simulink model "Motion_planner_Street_Drone"  (R2019b)
settings: Solver=FixedStepAuto  StartTime=0.0  StopTime=25  FixedStep=0.0075  MaxStep=1e-1  MinStep=1e-3  RelTol=1e-3  AbsTol=1e-4
InitFcn:
  | SD_init1
values from neighbouring files (symbols this model uses):
  cost = [2.71432892747 3.32441927977 3.79268757264 4.85642115368 6.12135035287 7.09825974303 9.57278659789 1.55754789407 1.51399555616 2.57723707661 3.8468529147 4.8336387623 ... (2430 elements, 1x2430)]    [matlab.mat]
  Front_brake = [0 2.2085352751 4.15209150797 6.12733711785 8.16604105928 9.79119154879 12.1808659635 14.1242630413 16.1155522836 18.1386900579 20.0839213981 22.1313006548 ... (68 elements, 34x2)]    [Front_brake.mat]
  N = size(X,1)    [curvature.m]
  obsx = [dx1 dx2 dx3 dx4]'    [dynamic_collison.m]    (also in dynamic_detection1.m = [x1 x2 x3 x4]')
  obsy = [dy1 dy2 dy3 dy4]'    [dynamic_collison.m]    (also in dynamic_detection1.m = [y1 y2 y3 y4]')
  x = obs_path(i,1)    [dynamic_collison.m]    (also in dynamic_detection1.m)
  X = [X]    [curvature.m]
  y = obs_path(i,2)    [dynamic_collison.m]    (also in dynamic_detection1.m)
undefined symbols (not defined in the file or in its folder): d, dfin, dini, Ki, Kp, L_0f, lookahead_time, lookahead_time_rev, Rear_brake, sigbuilder_block, steer_ratio, steer_sens, tfin, tini, TPS_0, xfin, Y, yfin, Z
libraries: sm_lib x290, nesl_utility x136, simulink x6, vrlib x2, powerlib_meascontrol x2
(part 13 of 14)

== system Motion_planner_Street_Drone/Trajectory Tracker/KM- StreetDrone/Street_Drone/Vehicle/RR_Wheel/For Validation ==
  Inputs : Inport
  Derivative : Derivative
  Integrator : Integrator
  Selector : Selector  InputPortWidth=40  IndexOptions=Index vector (dialog)  Indices=[3]  OutputSizes=1
  Selector1 : Selector  InputPortWidth=40  IndexOptions=Index vector (dialog)  Indices=[2]  OutputSizes=1
  Selector10 : Selector  InputPortWidth=40  IndexOptions=Index vector (dialog)  Indices=[28]  OutputSizes=1
  Selector11 : Selector  InputPortWidth=40  IndexOptions=Index vector (dialog)  Indices=[13]  OutputSizes=1
  Selector12 : Selector  InputPortWidth=40  IndexOptions=Index vector (dialog)  Indices=[5]  OutputSizes=1
  Selector2 : Selector  InputPortWidth=40  IndexOptions=Index vector (dialog)  Indices=[7]  OutputSizes=1
  Selector3 : Selector  InputPortWidth=40  IndexOptions=Index vector (dialog)  Indices=[1]  OutputSizes=1
  Selector4 : Selector  InputPortWidth=40  IndexOptions=Index vector (dialog)  Indices=[8]  OutputSizes=1
  Selector5 : Selector  InputPortWidth=40  IndexOptions=Index vector (dialog)  Indices=[11]  OutputSizes=1
  Selector6 : Selector  InputPortWidth=40  IndexOptions=Index vector (dialog)  Indices=[16]  OutputSizes=1
  Selector7 : Selector  InputPortWidth=40  IndexOptions=Index vector (dialog)  Indices=[17]  OutputSizes=1
  Selector8 : Selector  InputPortWidth=40  IndexOptions=Index vector (dialog)  Indices=[18]  OutputSizes=1
  Selector9 : Selector  InputPortWidth=40  IndexOptions=Index vector (dialog)  Indices=[24]  OutputSizes=1
  tag scope: RR_Fx=global, RR_Fy=global, RR_Fz=global, RR_Kappa=global, RR_My=global, RR_Re=global, RR_Vx=global, RR_alfa=global, RR_ax=global, RR_distance=global, RR_mu_x=global, RR_mu_y=global, RR_psi=global, RR_psidot=global, RR_tp=global
  wires:
  Selector12/1 -> [RR_My]
  Derivative/1 -> [RR_ax]
  Integrator/1 -> [RR_psi]
  Selector10/1 -> [RR_distance]
  Selector9/1 -> [RR_psidot], Integrator/1
  Selector8/1 -> [RR_mu_y]
  Selector7/1 -> [RR_mu_x]
  Selector6/1 -> [RR_tp]
  Selector5/1 -> [RR_Vx], Derivative/1
  Selector4/1 -> [RR_alfa]
  Selector3/1 -> [RR_Fx]
  Selector2/1 -> [RR_Kappa]
  Selector1/1 -> [RR_Fy]
  Selector/1 -> [RR_Fz]
  Selector11/1 -> [RR_Re]
  Inputs/1 -> Selector4/1, Selector2/1, Selector/1, Selector1/1, Selector3/1, Selector12/1, Selector5/1, Selector11/1, Selector6/1, Selector7/1, Selector8/1, Selector9/1, Selector10/1

== system Motion_planner_Street_Drone/Trajectory Tracker/KM- StreetDrone/Street_Drone/Vehicle/RR_Wheel/Non-moving road ==
  omega2 : Constant  Value=zeros(18,1)
  road : Outport
  wires:
  omega2/1 -> road/1

== system Motion_planner_Street_Drone/Trajectory Tracker/KM- StreetDrone/Street_Drone/Vehicle/RR_Wheel/Scaling factors ==
  s_LKX : Constant  Value=LKX
  s_LKY : Constant  Value=LKY
  s_LKYC : Constant  Value=LKYC
  s_LKZC : Constant  Value=LKZC
  s_LMUX : Constant  Value=LMUX
  s_LMUY : Constant  Value=LMUY
  s_LTR : Constant  Value=LTR
  scaling_vector : Mux  Inputs=7
  scaling : Outport
  wires:
  s_LMUX/1 -> scaling_vector/1
  s_LKX/1 -> scaling_vector/2
  s_LMUY/1 -> scaling_vector/3
  s_LKY/1 -> scaling_vector/4
  s_LKYC/1 -> scaling_vector/5
  s_LTR/1 -> scaling_vector/6
  s_LKZC/1 -> scaling_vector/7
  scaling_vector/1 -> scaling/1

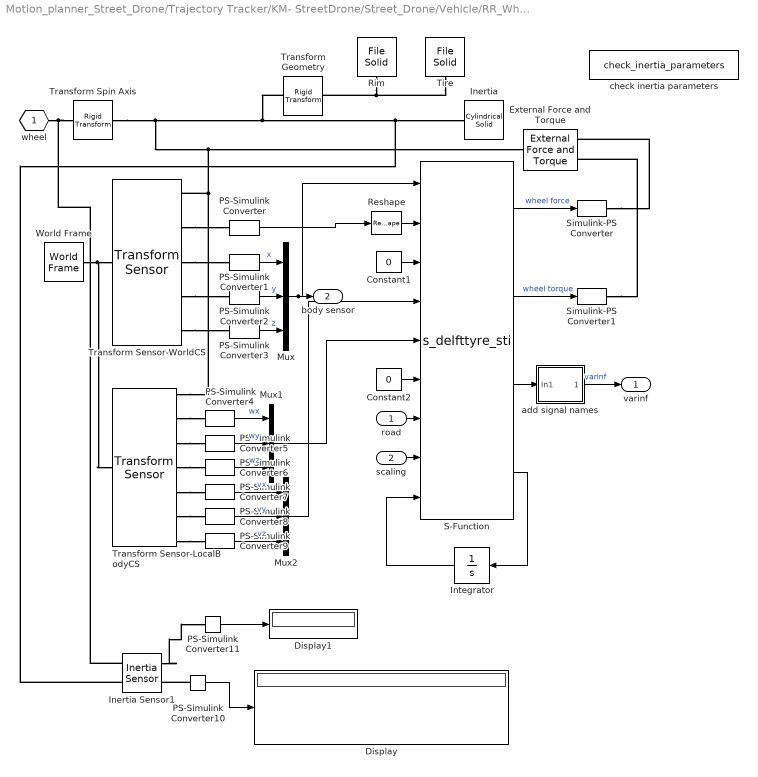
== system Motion_planner_Street_Drone/Trajectory Tracker/KM- StreetDrone/Street_Drone/Vehicle/RR_Wheel/SimMechanics2G Wheel + tyre ==
  road : Inport
  scaling : Inport  Port=2
  Constant1 : Constant  Value=0
  Constant2 : Constant  Value=0
  Display : Display
  Display1 : Display
  External Force and Torque : sm_lib/Forces and Torques/External Force and Torque  ForceResolutionFrame=AttachedFrame  EnableForceX=off  EnableForceY=off  EnableForceZ=off  EnableForce=on  TorqueResolutionFrame=AttachedFrame  EnableTorqueX=off  EnableTorqueY=off  EnableTorqueZ=off  EnableTorque=on
  Inertia : sm_lib/Body Elements/Cylindrical Solid  GraphicAmbientColor=[0.15 0.15 0.15 1.0]  BasedOnType=Density  CenterOfMass=[0 0 0]  CenterOfMassUnits=m  GraphicDiffuseColor=[0.2 0.8 1.0]  CylinderLength=0.001  CylinderLengthUnits=m  CylinderRadius=0.001  CylinderRadiusUnits=m  Density=1000  DensityUnits=kg/(m^3)  DoExposeReferenceFrame=on  GraphicEmissiveColor=[0.0 0.0 0.0 1.0]  ExportEntireGeometry=off  SerializedFrames=<Frames/>  MarkerShape=Sphere  MarkerSize=10  GraphicType=FromGeometry  InertiaType=Custom  Mass=mass  MassUnits=kg  MomentsOfInertia=[Imat(1,1) Imat(2,2) Imat(3,3)]  MomentsOfInertiaUnits=kg*m^2  GraphicOpacity=1.0  ProductsOfInertia=[0 0 0]  ProductsOfInertiaUnits=kg*m^2  GraphicShininess=75  GraphicSpecularColor=[0.5 0.5 0.5 1.0]  GraphicVisPropType=SimpleVisualProperties
  Inertia Sensor1 : sm_lib/Body Elements/Inertia Sensor  SensorExtent=BodyGroup  SpanWeldJoints=off  ExcludeGroundedBodies=off  MeasurementFrame=Custom  SenseMass=on  SenseCenterOfMass=off  SenseInertiaMatrix=on  SenseCenteredInertiaMatrix=off  SensePrincipalInertiaMatrix=off  SenseRotationMatrix=off  GraphicType=PrincipalInertiaFrame  PrincipalInertiaFrameSize=20  GraphicVisPropType=SimpleVisualProperties  GraphicDiffuseColor=[0.5 0.5 0.5]  GraphicSpecularColor=[0.5 0.5 0.5 1.0]  GraphicAmbientColor=[0.15 0.15 0.15 1.0]  GraphicEmissiveColor=[0.0 0.0 0.0 1.0]  GraphicShininess=75  GraphicOpacity=1.0
      settings: SourceProductBaseCode=MS
  Integrator : Integrator  InitialCondition=zeros(1,40)
  Mux : Mux  Inputs=3
  Mux1 : Mux  Inputs=3
  Mux2 : Mux  Inputs=3
  PS-Simulink Converter{,1..9} (10 alike) : nesl_utility/PS-Simulink Converter  PhysicalDomain=network_engine_domain  SubClassName=ps_output  LeftPortType=input  RightPortType=output  PseudoPeriodic=off  Frequencies=[]  Unit=1  AffineConversion=off
  PS-Simulink Converter10 : nesl_utility/PS-Simulink Converter  PhysicalDomain=network_engine_domain  SubClassName=ps_output  LeftPortType=input  RightPortType=output  PseudoPeriodic=off  Frequencies=[]  Unit=inherit  AffineConversion=off
  PS-Simulink Converter11 : nesl_utility/PS-Simulink Converter  PhysicalDomain=network_engine_domain  SubClassName=ps_output  LeftPortType=input  RightPortType=output  PseudoPeriodic=off  Frequencies=[]  Unit=inherit  AffineConversion=off
  Reshape : Reshape
  Rim : sm_lib/Body Elements/File Solid  ExtGeomFileName=D:\Project\PATH PLANNER STREET DRONE - 618341\CAD geometry\Rim_Back.stl  UnitType=Custom  ExtGeomFileUnits=mm  StepReaderType=HEX  ExportEntireGeometry=off  InertiaType=Custom  Mass=0  MassUnits=kg  CenterOfMass=[0 0 0]  CenterOfMassUnits=m  MomentsOfInertia=[0 0 0]  MomentsOfInertiaUnits=kg*m^2  ProductsOfInertia=[0 0 0]  ProductsOfInertiaUnits=kg*m^2  BasedOnType=Density  Density=1000  DensityUnits=kg/(m^3)  DoExposeReferenceFrame=on  SerializedFrames=<Frames/>  GraphicType=FromGeometry  MarkerShape=Sphere  MarkerSize=10  MarkerSizeUnits=m  GraphicVisPropType=SimpleVisualProperties  GraphicDiffuseColor=[0.8 0.8 0.8]  GraphicSpecularColor=[0.5 0.5 0.5 1.0]  GraphicAmbientColor=[0.15 0.15 0.15 1.0]  GraphicEmissiveColor=[0.0 0.0 0.0 1.0]  GraphicShininess=75  GraphicOpacity=1.0
  S-Function : S-Function  FunctionName=s_delfttyre_sti  Parameters=iswtch idtyre idroad tpfname_dummy rdfname typarr  SFunctionDeploymentMode=off  EnableBusSupport=off
  Simulink-PS Converter : nesl_utility/Simulink-PS Converter  PhysicalDomain=network_engine_domain  SubClassName=ps_input  LeftPortType=input  RightPortType=output  PseudoPeriodic=off  Frequencies=[]  NoiseDistribution=none  NoiseParameters=[]  Unit=1  AffineConversion=off  FilteringAndDerivatives=zero  SimscapeFilterOrder=1  InputFilterTimeConstant=0.001  UdotUserProvided=1
  Simulink-PS Converter1 : nesl_utility/Simulink-PS Converter  PhysicalDomain=network_engine_domain  SubClassName=ps_input  LeftPortType=input  RightPortType=output  PseudoPeriodic=off  Frequencies=[]  NoiseDistribution=none  NoiseParameters=[]  Unit=1  AffineConversion=off  FilteringAndDerivatives=zero  SimscapeFilterOrder=1  InputFilterTimeConstant=0.001  UdotUserProvided=1
  Tire : sm_lib/Body Elements/File Solid  ExtGeomFileName=D:\Project\PATH PLANNER STREET DRONE - 618341\CAD geometry\Tire_Back.stl  UnitType=Custom  ExtGeomFileUnits=mm  StepReaderType=HEX  ExportEntireGeometry=off  InertiaType=Custom  Mass=0  MassUnits=kg  CenterOfMass=[0 0 0]  CenterOfMassUnits=m  MomentsOfInertia=[0 0 0]  MomentsOfInertiaUnits=kg*m^2  ProductsOfInertia=[0 0 0]  ProductsOfInertiaUnits=kg*m^2  BasedOnType=Density  Density=1000  DensityUnits=kg/(m^3)  DoExposeReferenceFrame=on  SerializedFrames=<Frames/>  GraphicType=FromGeometry  MarkerShape=Sphere  MarkerSize=10  MarkerSizeUnits=m  GraphicVisPropType=SimpleVisualProperties  GraphicDiffuseColor=[0.5 0.5 0.5]  GraphicSpecularColor=[0.5 0.5 0.5 1.0]  GraphicAmbientColor=[0.15 0.15 0.15 1.0]  GraphicEmissiveColor=[0.0 0.0 0.0 1.0]  GraphicShininess=75  GraphicOpacity=1.0
  Transform Geometry : sm_lib/Frames and Transforms/Rigid Transform  TranslationMethod=StandardAxis  TranslationStandardOffset=(1-2*fliplr)*0.125  TranslationLengthUnit=m  TranslationStandardAxis=+Y  TranslationCartesianOffset=[0 0 0]  TranslationROffset=0  TranslationROffsetUnits=m  TranslationZOffset=0  TranslationZOffsetUnits=m  TranslationThetaOffset=0  TranslationThetaOffsetUnits=deg  RotationMethod=StandardAxis  RotationAngleUnits=deg  RotationStandardAxis=+X  RotationAngle=fliplr*180-90  RotationArbitraryAxis=[0 0 1]  FollAlignAxisA=+X  BaseAlignAxisA=+Y  FollAlignAxisB=+Y  BaseAlignAxisB=+Z  RotationSequenceAxes=FollowerAxes  RotationSequence=XYX  RotationSequenceAngles=[0 0 0]  RotationSequenceAnglesUnits=deg  RotationMatrix=[1 0 0; 0 1 0; 0 0 1]
  Transform Sensor-LocalBodyCS : sm_lib/Frames and Transforms/Transform Sensor  MeasurementFrame=NonRotatingFollower  SenseAngle=off  SenseAxis=off  SenseAngle1=off  SenseAngle2=off  SenseAngle3=off  SenseQ=off  SenseR=off  SenseOmegaX=on  SenseOmegaY=on  SenseOmegaZ=on  SenseOmega1=off  SenseOmega2=off  SenseOmega3=off  SenseQDot=off  SenseRDot=off  SenseAlphaX=off  SenseAlphaY=off  SenseAlphaZ=off  SenseAlpha1=off  SenseAlpha2=off  SenseAlpha3=off  SenseQDDot=off  SenseRDDot=off  SenseX=off  SenseY=off  SenseZ=off  SenseRad=off  SenseAzim=off  SenseDist=off  SenseInc=off  SenseXDot=on  SenseYDot=on  SenseZDot=on  SenseRadDot=off  SenseAzimDot=off  SenseDistDot=off  SenseIncDot=off  SenseXDDot=off  SenseYDDot=off  SenseZDDot=off  SenseRadDDot=off  SenseAzimDDot=off  SenseDistDDot=off  SenseIncDDot=off
  Transform Sensor-WorldCS : sm_lib/Frames and Transforms/Transform Sensor  MeasurementFrame=World  SenseAngle=off  SenseAxis=off  SenseAngle1=off  SenseAngle2=off  SenseAngle3=off  SenseQ=off  SenseR=on  SenseOmegaX=off  SenseOmegaY=off  SenseOmegaZ=off  SenseOmega1=off  SenseOmega2=off  SenseOmega3=off  SenseQDot=off  SenseRDot=off  SenseAlphaX=off  SenseAlphaY=off  SenseAlphaZ=off  SenseAlpha1=off  SenseAlpha2=off  SenseAlpha3=off  SenseQDDot=off  SenseRDDot=off  SenseX=on  SenseY=on  SenseZ=on  SenseRad=off  SenseAzim=off  SenseDist=off  SenseInc=off  SenseXDot=off  SenseYDot=off  SenseZDot=off  SenseRadDot=off  SenseAzimDot=off  SenseDistDot=off  SenseIncDot=off  SenseXDDot=off  SenseYDDot=off  SenseZDDot=off  SenseRadDDot=off  SenseAzimDDot=off  SenseDistDDot=off  SenseIncDDot=off
  Transform Spin Axis : sm_lib/Frames and Transforms/Rigid Transform  TranslationMethod=None  TranslationStandardOffset=0  TranslationLengthUnit=m  TranslationStandardAxis=+Z  TranslationCartesianOffset=[0 0 0]  TranslationROffset=0  TranslationROffsetUnits=m  TranslationZOffset=0  TranslationZOffsetUnits=m  TranslationThetaOffset=0  TranslationThetaOffsetUnits=deg  RotationMethod=StandardAxis  RotationAngleUnits=deg  RotationStandardAxis=-X  RotationAngle=90  RotationArbitraryAxis=[0 0 1]  FollAlignAxisA=+X  BaseAlignAxisA=+Y  FollAlignAxisB=+Y  BaseAlignAxisB=+Z  RotationSequenceAxes=FollowerAxes  RotationSequence=XYX  RotationSequenceAngles=[0 0 0]  RotationSequenceAnglesUnits=deg  RotationMatrix=[1 0 0; 0 1 0; 0 0 1]
  World Frame : sm_lib/Frames and Transforms/World Frame
  add signal names : Subsystem
  check inertia parameters : M-S-Function  Priority=1  FunctionName=check_inertia_parameters  Parameters=tpfname1, rdfname1, typarr1  mask{tpfname1=tpfname_dummy, rdfname1=rdfname, typarr1=typarr}
      mask prompts: tpfname1 "Tyre Property File"; rdfname1 "Road Data File"; typarr1 "typarr"
      mask help: Checks Inertia parameters as calculated in mask
  wheel : PMIOPort  Side=Left
  varinf : Outport
  body sensor : Outport  Port=2
  wires:
  PS-Simulink Converter11/1 -> Display1/1
  PS-Simulink Converter10/1 -> Display/1
  Constant2/1 -> S-Function/6
  Mux2/1 -> S-Function/4
  Mux1/1 -> S-Function/5
  PS-Simulink Converter/1 -> Reshape/1
  S-Function/4 -> Integrator/1
  S-Function/3 -> add signal names/1(In1)
  add signal names/1(Out1) -> varinf/1  "varinf"
  road/1 -> S-Function/7
  scaling/1 -> S-Function/8
  Integrator/1 -> S-Function/9
  Constant1/1 -> S-Function/3
  PS-Simulink Converter1/1 -> Mux/1  "x"
  PS-Simulink Converter2/1 -> Mux/2  "y"
  PS-Simulink Converter3/1 -> Mux/3  "z"
  PS-Simulink Converter4/1 -> Mux1/1  "wx"
  PS-Simulink Converter5/1 -> Mux1/2  "wy"
  PS-Simulink Converter6/1 -> Mux1/3  "wz"
  PS-Simulink Converter7/1 -> Mux2/1  "vx"
  PS-Simulink Converter8/1 -> Mux2/2  "vy"
  PS-Simulink Converter9/1 -> Mux2/3  "vz"
  Mux/1 -> body sensor/1, S-Function/1
  S-Function/2 -> Simulink-PS Converter1/1  "wheel torque"
  S-Function/1 -> Simulink-PS Converter/1  "wheel force"
  Reshape/1 -> S-Function/2
  connections:
  Inertia Sensor1/RConn1 -- PS-Simulink Converter11/LConn1
  PS-Simulink Converter10/LConn1 -- Inertia Sensor1/RConn2
  Inertia Sensor1/LConn1 -- wheel/RConn1 -- Transform Spin Axis/RConn1
  Simulink-PS Converter1/RConn1 -- External Force and Torque/LConn2
  Simulink-PS Converter/RConn1 -- External Force and Torque/LConn1
  Transform Sensor-WorldCS/RConn2 -- PS-Simulink Converter/LConn1
  Transform Sensor-WorldCS/RConn3 -- PS-Simulink Converter1/LConn1
  Transform Sensor-WorldCS/RConn4 -- PS-Simulink Converter2/LConn1
  Transform Sensor-WorldCS/RConn5 -- PS-Simulink Converter3/LConn1
  Transform Sensor-LocalBodyCS/RConn2 -- PS-Simulink Converter4/LConn1
  Transform Sensor-LocalBodyCS/RConn3 -- PS-Simulink Converter5/LConn1
  Transform Sensor-LocalBodyCS/RConn4 -- PS-Simulink Converter6/LConn1
  Transform Sensor-LocalBodyCS/RConn5 -- PS-Simulink Converter7/LConn1
  Transform Sensor-LocalBodyCS/RConn6 -- PS-Simulink Converter8/LConn1
  Transform Sensor-LocalBodyCS/RConn7 -- PS-Simulink Converter9/LConn1
  Tire/RConn1 -- Rim/RConn1 -- Transform Geometry/RConn1
  Inertia Sensor1/LConn2 -- Transform Geometry/LConn1 -- External Force and Torque/RConn1 -- Transform Sensor-LocalBodyCS/RConn1 -- Transform Sensor-WorldCS/RConn1 -- Transform Spin Axis/LConn1 -- Inertia/RConn1
  Transform Sensor-LocalBodyCS/LConn1 -- World Frame/RConn1 -- Transform Sensor-WorldCS/LConn1

== system Motion_planner_Street_Drone/Trajectory Tracker/KM- StreetDrone/Street_Drone/Inputs/Velocity/Normal_manoever/Forward ==
  Demux : Demux  Tag=STV Demux  Outputs=1
  FromWs : FromWorkspace  Tag=STV FromWs  VariableName=tuvar  SampleTime=0
      SigBuilderData=|
      | common.afterFinalStr = 'Extrapolate'
      | common.sampleTime = 0
      | dataSet.timeRange = [0 60]
      | dataSet.name = 'Group 1'
      | sbobj.Groups.Name = 'Group 1'
      | sbobj.Groups.Signals.Name = 'Signal 1'
      | sbobj.Groups.Signals.XData = [0 1 6 13.5 18.5 20 32 32 35 40 60]
      | sbobj.Groups.Signals.YData = [0 0 8.333333 8.3 0 0 21.1 20 20 20 20]
      | sbobj.Groups.TimeRange = [0 60]
  Signal 1 : Outport  Tag=STV Outport
  wires:
  FromWs/1 -> Demux/1
  Demux/1 -> Signal 1/1

== system Motion_planner_Street_Drone/Trajectory Tracker/KM- StreetDrone/Street_Drone/Inputs/Velocity/Normal_manoever/Reverse ==
  Demux : Demux  Tag=STV Demux  Outputs=1
  FromWs : FromWorkspace  Tag=STV FromWs  VariableName=tuvar  SampleTime=0
      SigBuilderData=|
      | common.afterFinalStr = 'Extrapolate'
      | common.sampleTime = 0
      | dataSet.timeRange = [0 60]
      | dataSet.name = 'Group 1'
      | sbobj.Groups.Name = 'Group 1'
      | sbobj.Groups.Signals.Name = 'Signal 1'
      | sbobj.Groups.Signals.XData = [0 1 6 13.5 18.5 20 32 32 35 40 60]
      | sbobj.Groups.Signals.YData = [0 0 2.7778 2.7778 0 0 21.1 20 20 20 20]
      | sbobj.Groups.TimeRange = [0 60]
  Signal 1 : Outport  Tag=STV Outport
  wires:
  Demux/1 -> Signal 1/1
  FromWs/1 -> Demux/1

== system Motion_planner_Street_Drone/Trajectory Tracker/KM- StreetDrone/Street_Drone/Results1/Fx/Calculated/Torque_inertia ==
  RL : Subsystem
  RR : Subsystem

== system Motion_planner_Street_Drone/Trajectory Tracker/KM- StreetDrone/Street_Drone/Results1/Fx/Calculated/Whole_vehicle ==
  Product : Product
  To Workspace3 : ToWorkspace  VariableName=Calc_Fx_vehicle  SampleTime=-1
  wires:
  [mass] -> Product/2
  Product/1 -> To Workspace3/1
  [Act_Ax] -> Product/1

== system Motion_planner_Street_Drone/Trajectory Tracker/KM- StreetDrone/Street_Drone/Vehicle/FL_Wheel/SimMechanics2G Wheel + tyre/add signal names ==
  In1 : Inport
  Added for future extension : Terminator
  Bus Creator : BusCreator  Inputs=40
  Demux1 : Demux  Outputs=[ones(1,40) -1]
  Out1 : Outport
  wires:
  In1/1 -> Demux1/1
  Bus Creator/1 -> Out1/1  "varinf"
  Demux1/1 -> Bus Creator/1  "Fx"
  Demux1/2 -> Bus Creator/2  "Fy"
  Demux1/3 -> Bus Creator/3  "Fz"
  Demux1/4 -> Bus Creator/4  "Mx"
  Demux1/5 -> Bus Creator/5  "My"
  Demux1/6 -> Bus Creator/6  "Mz"
  Demux1/7 -> Bus Creator/7  "longitudinal_slip"
  Demux1/8 -> Bus Creator/8  "side_slip_angle"
  Demux1/9 -> Bus Creator/9  "inclination_angle"
  Demux1/10 -> Bus Creator/10  "turn_slip"
  Demux1/11 -> Bus Creator/11  "Vx"
  Demux1/12 -> Bus Creator/12  "_e12"
  Demux1/13 -> Bus Creator/13  "effective_rolling_radius"
  Demux1/14 -> Bus Creator/14  "vertical_deflection"
  Demux1/15 -> Bus Creator/15  "contact_length"
  Demux1/16 -> Bus Creator/16  "pneumatic_trail"
  Demux1/17 -> Bus Creator/17  "mu_x"
  Demux1/18 -> Bus Creator/18  "mu_y"
  Demux1/19 -> Bus Creator/19  "relaxation_length_x"
  Demux1/20 -> Bus Creator/20  "relaxation_length_y"
  Demux1/21 -> Bus Creator/21  "Vsx"
  Demux1/22 -> Bus Creator/22  "Vsy"
  Demux1/23 -> Bus Creator/23  "Vz"
  Demux1/24 -> Bus Creator/24  "psidot"
  Demux1/25 -> Bus Creator/25  "_e25"
  Demux1/26 -> Bus Creator/26  "_e26"
  Demux1/27 -> Bus Creator/27  "_e27"
  Demux1/28 -> Bus Creator/28  "travelled_distance"
  Demux1/29 -> Bus Creator/29  "_e29"
  Demux1/30 -> Bus Creator/30  "_e30"
  Demux1/31 -> Bus Creator/31  "xcp"
  Demux1/32 -> Bus Creator/32  "ycp"
  Demux1/33 -> Bus Creator/33  "zcp"
  Demux1/34 -> Bus Creator/34  "nx"
  Demux1/35 -> Bus Creator/35  "ny"
  Demux1/36 -> Bus Creator/36  "nz"
  Demux1/37 -> Bus Creator/37  "eff_plane_height"
  Demux1/38 -> Bus Creator/38  "eff_plane_angle"
  Demux1/39 -> Bus Creator/39  "eff_plane_curvature"
  Demux1/40 -> Bus Creator/40  "eff_plane_banking"
  Demux1/41 -> Added for future extension/1

== system Motion_planner_Street_Drone/Trajectory Tracker/KM- StreetDrone/Street_Drone/Vehicle/FR_Wheel/SimMechanics2G Wheel + tyre/add signal names ==
  In1 : Inport
  Added for future extension : Terminator
  Bus Creator : BusCreator  Inputs=40
  Demux1 : Demux  Outputs=[ones(1,40) -1]
  Out1 : Outport
  wires:
  Demux1/41 -> Added for future extension/1
  Demux1/40 -> Bus Creator/40  "eff_plane_banking"
  Demux1/39 -> Bus Creator/39  "eff_plane_curvature"
  Demux1/38 -> Bus Creator/38  "eff_plane_angle"
  Demux1/37 -> Bus Creator/37  "eff_plane_height"
  Demux1/36 -> Bus Creator/36  "nz"
  Demux1/35 -> Bus Creator/35  "ny"
  Demux1/34 -> Bus Creator/34  "nx"
  Demux1/33 -> Bus Creator/33  "zcp"
  Demux1/32 -> Bus Creator/32  "ycp"
  Demux1/31 -> Bus Creator/31  "xcp"
  Demux1/30 -> Bus Creator/30  "_e30"
  Demux1/29 -> Bus Creator/29  "_e29"
  Demux1/28 -> Bus Creator/28  "travelled_distance"
  Demux1/27 -> Bus Creator/27  "_e27"
  Demux1/26 -> Bus Creator/26  "_e26"
  Demux1/25 -> Bus Creator/25  "_e25"
  Demux1/24 -> Bus Creator/24  "psidot"
  Demux1/23 -> Bus Creator/23  "Vz"
  Demux1/22 -> Bus Creator/22  "Vsy"
  Demux1/21 -> Bus Creator/21  "Vsx"
  Demux1/20 -> Bus Creator/20  "relaxation_length_y"
  Demux1/19 -> Bus Creator/19  "relaxation_length_x"
  Demux1/18 -> Bus Creator/18  "mu_y"
  Demux1/17 -> Bus Creator/17  "mu_x"
  Demux1/16 -> Bus Creator/16  "pneumatic_trail"
  Demux1/15 -> Bus Creator/15  "contact_length"
  Demux1/14 -> Bus Creator/14  "vertical_deflection"
  Demux1/13 -> Bus Creator/13  "effective_rolling_radius"
  Demux1/12 -> Bus Creator/12  "_e12"
  Demux1/11 -> Bus Creator/11  "Vx"
  Demux1/10 -> Bus Creator/10  "turn_slip"
  Demux1/9 -> Bus Creator/9  "inclination_angle"
  Demux1/8 -> Bus Creator/8  "side_slip_angle"
  Demux1/7 -> Bus Creator/7  "longitudinal_slip"
  Demux1/6 -> Bus Creator/6  "Mz"
  Demux1/5 -> Bus Creator/5  "My"
  Demux1/4 -> Bus Creator/4  "Mx"
  Demux1/3 -> Bus Creator/3  "Fz"
  Demux1/2 -> Bus Creator/2  "Fy"
  Demux1/1 -> Bus Creator/1  "Fx"
  Bus Creator/1 -> Out1/1  "varinf"
  In1/1 -> Demux1/1

== system Motion_planner_Street_Drone/Trajectory Tracker/KM- StreetDrone/Street_Drone/Vehicle/RL_Wheel/SimMechanics2G Wheel + tyre/add signal names ==
  In1 : Inport
  Added for future extension : Terminator
  Bus Creator : BusCreator  Inputs=40
  Demux1 : Demux  Outputs=[ones(1,40) -1]
  Out1 : Outport
  wires:
  Demux1/41 -> Added for future extension/1
  Demux1/40 -> Bus Creator/40  "eff_plane_banking"
  Demux1/39 -> Bus Creator/39  "eff_plane_curvature"
  Demux1/38 -> Bus Creator/38  "eff_plane_angle"
  Demux1/37 -> Bus Creator/37  "eff_plane_height"
  Demux1/36 -> Bus Creator/36  "nz"
  Demux1/35 -> Bus Creator/35  "ny"
  Demux1/34 -> Bus Creator/34  "nx"
  Demux1/33 -> Bus Creator/33  "zcp"
  Demux1/32 -> Bus Creator/32  "ycp"
  Demux1/31 -> Bus Creator/31  "xcp"
  Demux1/30 -> Bus Creator/30  "_e30"
  Demux1/29 -> Bus Creator/29  "_e29"
  Demux1/28 -> Bus Creator/28  "travelled_distance"
  Demux1/27 -> Bus Creator/27  "_e27"
  Demux1/26 -> Bus Creator/26  "_e26"
  Demux1/25 -> Bus Creator/25  "_e25"
  Demux1/24 -> Bus Creator/24  "psidot"
  Demux1/23 -> Bus Creator/23  "Vz"
  Demux1/22 -> Bus Creator/22  "Vsy"
  Demux1/21 -> Bus Creator/21  "Vsx"
  Demux1/20 -> Bus Creator/20  "relaxation_length_y"
  Demux1/19 -> Bus Creator/19  "relaxation_length_x"
  Demux1/18 -> Bus Creator/18  "mu_y"
  Demux1/17 -> Bus Creator/17  "mu_x"
  Demux1/16 -> Bus Creator/16  "pneumatic_trail"
  Demux1/15 -> Bus Creator/15  "contact_length"
  Demux1/14 -> Bus Creator/14  "vertical_deflection"
  Demux1/13 -> Bus Creator/13  "effective_rolling_radius"
  Demux1/12 -> Bus Creator/12  "_e12"
  Demux1/11 -> Bus Creator/11  "Vx"
  Demux1/10 -> Bus Creator/10  "turn_slip"
  Demux1/9 -> Bus Creator/9  "inclination_angle"
  Demux1/8 -> Bus Creator/8  "side_slip_angle"
  Demux1/7 -> Bus Creator/7  "longitudinal_slip"
  Demux1/6 -> Bus Creator/6  "Mz"
  Demux1/5 -> Bus Creator/5  "My"
  Demux1/4 -> Bus Creator/4  "Mx"
  Demux1/3 -> Bus Creator/3  "Fz"
  Demux1/2 -> Bus Creator/2  "Fy"
  Demux1/1 -> Bus Creator/1  "Fx"
  Bus Creator/1 -> Out1/1  "varinf"
  In1/1 -> Demux1/1

== system Motion_planner_Street_Drone/Trajectory Tracker/KM- StreetDrone/Street_Drone/Vehicle/RR_Wheel/SimMechanics2G Wheel + tyre/add signal names ==
  In1 : Inport
  Added for future extension : Terminator
  Bus Creator : BusCreator  Inputs=40
  Demux1 : Demux  Outputs=[ones(1,40) -1]
  Out1 : Outport
  wires:
  In1/1 -> Demux1/1
  Bus Creator/1 -> Out1/1  "varinf"
  Demux1/1 -> Bus Creator/1  "Fx"
  Demux1/2 -> Bus Creator/2  "Fy"
  Demux1/3 -> Bus Creator/3  "Fz"
  Demux1/4 -> Bus Creator/4  "Mx"
  Demux1/5 -> Bus Creator/5  "My"
  Demux1/6 -> Bus Creator/6  "Mz"
  Demux1/7 -> Bus Creator/7  "longitudinal_slip"
  Demux1/8 -> Bus Creator/8  "side_slip_angle"
  Demux1/9 -> Bus Creator/9  "inclination_angle"
  Demux1/10 -> Bus Creator/10  "turn_slip"
  Demux1/11 -> Bus Creator/11  "Vx"
  Demux1/12 -> Bus Creator/12  "_e12"
  Demux1/13 -> Bus Creator/13  "effective_rolling_radius"
  Demux1/14 -> Bus Creator/14  "vertical_deflection"
  Demux1/15 -> Bus Creator/15  "contact_length"
  Demux1/16 -> Bus Creator/16  "pneumatic_trail"
  Demux1/17 -> Bus Creator/17  "mu_x"
  Demux1/18 -> Bus Creator/18  "mu_y"
  Demux1/19 -> Bus Creator/19  "relaxation_length_x"
  Demux1/20 -> Bus Creator/20  "relaxation_length_y"
  Demux1/21 -> Bus Creator/21  "Vsx"
  Demux1/22 -> Bus Creator/22  "Vsy"
  Demux1/23 -> Bus Creator/23  "Vz"
  Demux1/24 -> Bus Creator/24  "psidot"
  Demux1/25 -> Bus Creator/25  "_e25"
  Demux1/26 -> Bus Creator/26  "_e26"
  Demux1/27 -> Bus Creator/27  "_e27"
  Demux1/28 -> Bus Creator/28  "travelled_distance"
  Demux1/29 -> Bus Creator/29  "_e29"
  Demux1/30 -> Bus Creator/30  "_e30"
  Demux1/31 -> Bus Creator/31  "xcp"
  Demux1/32 -> Bus Creator/32  "ycp"
  Demux1/33 -> Bus Creator/33  "zcp"
  Demux1/34 -> Bus Creator/34  "nx"
  Demux1/35 -> Bus Creator/35  "ny"
  Demux1/36 -> Bus Creator/36  "nz"
  Demux1/37 -> Bus Creator/37  "eff_plane_height"
  Demux1/38 -> Bus Creator/38  "eff_plane_angle"
  Demux1/39 -> Bus Creator/39  "eff_plane_curvature"
  Demux1/40 -> Bus Creator/40  "eff_plane_banking"
  Demux1/41 -> Added for future extension/1

== system Motion_planner_Street_Drone/Trajectory Tracker/KM- StreetDrone/Street_Drone/Results1/Fx/Calculated/Torque_inertia/RL ==
  Add : Sum
  Add1 : Sum  Inputs=+-
  Divide2 : Product  Inputs=*/
  Divide3 : Product  Inputs=*/
  Ie : Constant  Value=0.0226
  Iw : Constant  Value=0.4665
  Product2 : Product
  Product3 : Product
  Scope1 : Scope
  Scope3 : Scope
  Scope4 : Scope
  To Workspace1 : ToWorkspace  VariableName=calc_Fx_RL  SampleTime=-1
  tag scope: Iner_loss_L=global
  wires:
  Add/1 -> Product2/1
  Add1/1 -> To Workspace1/1, Scope1/1
  Divide3/1 -> Add1/2, [Iner_loss_L], Scope4/1
  Product3/1 -> Divide3/2
  Ie/1 -> Add/1
  [Me_Pt] -> Divide2/1
  [RL_Re] -> Divide2/2
  Iw/1 -> Add/2
  [RL_Re] -> Product3/1
  [Act_Ax] -> Product2/2
  Product2/1 -> Divide3/1
  Divide2/1 -> Add1/1, Scope3/1
  [RL_Re] -> Product3/2

== system Motion_planner_Street_Drone/Trajectory Tracker/KM- StreetDrone/Street_Drone/Results1/Fx/Calculated/Torque_inertia/RR ==
  Add2 : Sum
  Add3 : Sum  Inputs=+-
  Divide1 : Product  Inputs=*/
  Divide4 : Product  Inputs=*/
  Ie_R : Constant  Value=0.0226
  Iw_R : Constant  Value=0.4665
  Product1 : Product
  Product4 : Product
  Scope2 : Scope
  Scope5 : Scope
  Scope6 : Scope
  To Workspace2 : ToWorkspace  VariableName=calc_Fx_RR  SampleTime=-1
  tag scope: Iner_loss_R=global
  wires:
  Add2/1 -> Product1/1
  [Me_Pt] -> Divide1/1
  Iw_R/1 -> Add2/2
  Product1/1 -> Divide4/1
  [RR_Re] -> Divide1/2
  [Act_Ax] -> Product1/2
  Ie_R/1 -> Add2/1
  [RR_Re] -> Product4/1
  Add3/1 -> To Workspace2/1, Scope2/1
  Divide1/1 -> Add3/1, Scope6/1
  [RR_Re] -> Product4/2
  Divide4/1 -> Add3/2, Scope5/1, [Iner_loss_R]
  Product4/1 -> Divide4/2

== matlab function Motion_planner_Street_Drone/Trajectory Tracker/ Lateral Controller/Rev_Controller1/MATLAB Function1 ==
  data: data input; u input; y output
function y = fcn(data, u)
if u==-1
    y=0;
else
y = data(u);


end

== matlab function Motion_planner_Street_Drone/Motion_planning/Motion_Planner/MATLAB Function ==
  data: start input; goal input; obsc input; obsx input; obsy input; cost input; d input; dfin input; dini input; t input; tfin input; tini input; x input; xfin input; y input; yfin input; toctime output; path output; mode input; d_dobst input; stop output; steer output
    function [ toctime,path,stop,steer] = motionPlanning(start,goal,obsc,obsx,obsy,cost,d,dfin,dini,t,tfin,tini,x,xfin,y,yfin,mode, d_dobst)
%% This is motion planning system. In this system based on the mode it select the A_star or A_star2
%#codegen
tictime     =   tic;  
%predifine the stete of the vehicle
% i_state   =   struct('x',0,'y',0,'t',0,'d',0);
% f_state   =   struct('x',0,'y',0,'t',0);
%% Parking Maneuver
%  if mode==3 
% i_state.x   = 86.9;    %[m]
% i_state.y  =0;         %[m]
% i_state.t   =  0;      %[degrees] have to be a discreet theta config
% i_state.d   =   0 ;    %Initial Steering angle
% f_state.x   = goal(1); %[m]
% f_state.y   = goal(2);   %[m]
% f_state.t   = goal(3);
%   stop=3;
%  [loopcheck,o, c, cc, cur, t_pred, i_state, x, y, t_predxy, t_x, t_xa, t_y, t_ya,  t_dir, t_count, t_hcost]=A_star2(cost,d,dfin,dini,t,tfin,tini,x,xfin,y,yfin,obsc,obsx,obsy,i_state,f_state)
% 
%  else
 %% Navigation Maneuver
i_state.x   = start(1);    %[m]
i_state.y  =start(2);     %[m]
i_state.t   =  round(rad2deg(start(3))/3)*3;     %[degrees] have to be a discreet theta config
i_state.d   =   0 ;
f_state.x   = goal(1);    %[m]
f_state.y  =goal(2);     %[m]
f_state.t  =goal(3);      %[degrees] have to be a discreet theta config
 %i_state.d   =   0 ;
 %% dynamic obstacle shape
 x_dobst=d_dobst(1);
 y_dobst=d_dobst(2);
 thetad=d_dobst(3);
 lz= 2;     %length
 wz= 1.5;   %width
 dt1 = (180/pi*thetad)+90+atand(wz/lz); % Angle of Vector 1
 dt2 = (180/pi*thetad)-90-atand(wz/lz); % Angle of Vector 2
 dt3 = (180/pi*thetad)-atand(wz/lz); % Angle of Vector 3
 dt4 = (180/pi*thetad)+atand(wz/lz); % Angle of Vector 4

dl= hypot(wz/2,lz/2);
dx1= x_dobst + dl*cosd(dt1);
dy1=   y_dobst + dl*sind(dt1);
dx2=  x_dobst + dl*cosd(dt2);
dy2=   y_dobst + (dl)*sind(dt2);
dx3= x_dobst + dl*cosd(dt3);
dy3=   y_dobst + (dl)*sind(dt3);
dx4= x_dobst + dl*cosd(dt4);
dy4=   y_dobst+ dl*sind(dt4);
%dynamic obstacle points
dobsx = [dx1 dx2 dx3 dx4];
dobsy = [dy1 dy2 dy3 dy4];
stop=2;

 [ o, c, cc, cur, t_pred, x, y, t_predxy, t_x, t_xa, t_y, t_ya,  t_dir, t_count, t_hcost ]=A_star(cost,d,dfin,dini,t,tfin,tini,x,xfin,y,yfin,obsc,obsx,obsy,i_state,f_state,dobsx,dobsy);

 
%  end
toctime=((toc(tictime)));
  

%% In this section path is extracted from C-list
indexp  =   c(cc);
indexmp =   t_pred(indexp);
% Creating arrays to store path info.
pathx1=zeros(21,20);
pathy1=zeros(21,20);
pathdir1=zeros(1,20);
i=0;

pathtfin1=zeros(21,20);
pathdelta=zeros(21,20);

% Exctracting path information from tree
while (t_x(indexp)~= i_state.x || t_y(indexp) ~= i_state.y)&& ~isnan(indexmp)
    xp  =   x(:,indexmp);
    yp  =   y(:,indexmp);
    thetap  =   t(:,indexmp);
    deltap=d(:,indexmp);
    dirp    =   t_dir(indexp);
    pred_index  =   t_predxy(indexp);
    if dirp==1
        xp= xp+t_xa(pred_index);
        yp= yp+t_ya(pred_index);
       % theta=thetap;
    else
        xp=xp-xp(length(xp))+t_xa(pred_index);
        yp=yp-yp(length(yp))+t_ya(pred_index);
        xp=flip(xp);
        yp=flip(yp);
        thetap=flip(thetap);
        deltap=flip(deltap);
    end
    i   =   i+1;            % Array index
    pathx1(:,i)  =   xp;     % Storing path information                                                             
    pathy1(:,i)  =   yp;
    pathdir1(i) =   dirp;
    pathtfin1(:,i)=thetap;
    pathdelta(:,i)=deltap;

   % pathtfin =   thetap;
    indexp      =   t_predxy(indexp);
    indexmp     =   t_pred(indexp);
end


% toctime=((toc(tictime))) % Finding the computational time
 path=nan(1000,4);
 steer=nan(1000,1);
 k=1;
for m=i:-1:1
    for j=1:21
        path(k,1)=pathx1(j,m);
        path(k,2)=pathy1(j,m);
       path(k,3)=pathtfin1(j,m);
        path(k,4)=pathdir1(:,m);
        steer(k,1)=pathdelta(j,m);
        k=k+1;
    end
end
%% to plot the path
figure(1)
plot(path(:,1),path(:,2),'Linewidth',2);
xlabel('X [meters]');
ylabel('Y [meters]');
xlim([-10 170]);
ylim([-10 10]);
title('Path generated by planner for lane change');
hold on
end

== matlab function Motion_planner_Street_Drone/Trajectory Tracker/ Lateral Controller/Fwd_Controller/Embedded MATLAB Function ==
  data: path input; point input; dist output; npoints input; pos output; idx2 output; idx1 input; alpha output; b_dist output; worldchanged input
function [dist,pos,idx2,alpha,b_dist] = dist2path(path,point,npoints,idx1,worldchanged)
%#eml
 select = ~isnan(path(1,:));
path1=path(select);
persistent a b c idx mdist dist_sgn

a=[0 0 0]';
b=[0 0 0]';
c=[0 0 0]';
pos=[0 0 0]';

b_dist=[0 0 0]';
mdist=[0];
idx=0;
if worldchanged==0
idx=idx1;
end
alpha=[0];

%Determination of idx_min and idx_max : plage de [idx-npoints,idx+npoints]
%npoints=10
if idx<0
    idx_min=1;
    idx_max=length(path1);
else
    idx_min=max(1,idx-npoints);
    idx_max=min(length(path1),idx+npoints);
end

% idx_min_dist=0;
min_dist=1e8;

%Determination of the shortest path to the closest reference point
for i=idx_min:idx_max
    mdist=norm(path(:,i) - point);  % Distance viewpoint to reference path for all reference points
    if mdist<min_dist               % If distance is smaller than previous distance
        idx=i;                      % Shortest path is reference point i            
        min_dist=mdist;         	% Shortest distance is updated 
        pos=path(:,i) ;         	% Reference point on reference path is updated.
        
    end
end

%Indice   Keeping reference point inside the reference path
idx=max(idx,2);
idx=min(idx,length(path1)-1);


for i=idx-1:idx      
    a=path(:,i+1)-path(:,i);    %[dx dy dz] of distance between minimal ref point and previous point
    b=point-path(:,i);          % distance between reaction point and reference point
    
    b_dist=b;
    alpha=dot(a,b)/dot(a,a);    %product vectors a,b /  product vectors a,a -> rapport distance a et projection de b sur a
    dist=norm(b-alpha*a);       %distance avec la trajectoire droite entre les deux points
    
    if alpha > 0 && alpha < 1 && dist < min_dist %Le vehicule est avant le point vise  
        min_dist=dist;  %Distance mini
        pos=path(:,i)+alpha*a;  %point reellement vise
        
        idx=i;              
        c=cross(a,b);       %produit vectoriel  
        dist_sgn=sign(c(3));        %signe du produit vectoriel au niveau de Z
    end
end

a= path(:,idx+1) - path(:,idx);
b= point - pos;
c= cross(a,b);
dist_sgn=sign(c(3));

dist= min_dist*dist_sgn;
idx2=idx;

== matlab function Motion_planner_Street_Drone/Goal_check/MATLAB Function ==
  data: goal input; stop output; x input; y input
function stop  = fcn(goal,x,y)
%to check the vehicle reach the goal point

if abs(goal(1,1)-x)<0.1 && abs(goal(1,2)-y)<0.1
   stop=1;
else
    stop=0;
end

== matlab function Motion_planner_Street_Drone/Trajectory Tracker/ Lateral Controller/Rev_Controller1/Embedded MATLAB Function ==
  settings: updateMethod=DISCRETE
  data: path input; point input; dist output; npoints input; pos output; idx2 output; idx1 input; alpha output; b_dist output; worldchanged input
function [dist,pos,idx2,alpha,b_dist] = dist2path(path,point,npoints,idx1, worldchanged)
%#eml
 select = ~isnan(path(1,:));
path1=path(select);
persistent a b c idx mdist dist_sgn

a=[0 0 0]';
b=[0 0 0]';
c=[0 0 0]';
pos=[0 0 0]';
b_dist=[0 0 0]';
mdist=[0];

if worldchanged==1
idx=0;
else
    idx=idx1;
end
alpha=[0];

%Determination of idx_min and idx_max : plage de [idx-npoints,idx+npoints]
%npoints=10
if idx<0
    idx_min=1;
    idx_max=length(path1);
else
    idx_min=max(1,idx-npoints);
    idx_max=min(length(path1),idx+npoints);
end

% idx_min_dist=0;
min_dist=1e8;

%Determination of the shortest path to the closest reference point
for i=idx_min:idx_max
    mdist=norm(path(:,i) - point);  % Distance viewpoint to reference path for all reference points
    if mdist<min_dist               % If distance is smaller than previous distance
        idx=i;                      % Shortest path is reference point i            
        min_dist=mdist;         	% Shortest distance is updated 
        pos=path(:,i);          	% Reference point on reference path is updated.
    end
end

%Indice   Keeping reference point inside the reference path
idx=max(idx,2);
idx=min(idx,length(path1)-1);


for i=idx-1:idx      
    a=path(:,i+1)-path(:,i);    %[dx dy dz] of distance between minimal ref point and previous point
    b=point-path(:,i);          % distance between reaction point and reference point
    
    b_dist=b;
    alpha=dot(a,b)/dot(a,a);    %product vectors a,b /  product vectors a,a -> rapport distance a et projection de b sur a
    dist=norm(b-alpha*a);       %distance avec la trajectoire droite entre les deux points
    
    if alpha > 0 && alpha < 1 && dist < min_dist %Le vehicule est avant le point vise  
        min_dist=dist;  %Distance mini
        pos=path(:,i)+alpha*a;  %point reellement vise
        idx=i;              
        c=cross(a,b);       %produit vectoriel  
        dist_sgn=sign(c(3));        %signe du produit vectoriel au niveau de Z
    end
end

a= path(:,idx+1) - path(:,idx);
b= point - pos;
c= cross(a,b);
dist_sgn=sign(c(3));

dist= min_dist*dist_sgn;
idx2=idx;

== matlab function Motion_planner_Street_Drone/Motion_planning/Velocity_profile/Waypoints ==
  data: path1 input; path_input output; velocity output; goal output; vel1 output; path_tf output; mode input; V_in input
 function [path_input,velocity,goal,vel1,path_tf]  = fcn(path1, mode, V_in)
%% Velocity Profile generation
%#eml
goal=nan(1,2);
 extx=nan(2000,1);
 exty=nan(2000,1);
 vel1=nan(1,2000);
%  %velocity profile for reverse path
% if mode==-1
%     dir=-1;
%  index=find((path1(:,4)==-1));
%   index2=length(index);
%  path=nan(index2*5,3);
%  path_input=nan(2000,3);
%  Length=nan(1,2000);
%  velocity=nan(1,2000);
%  path_tf=nan(1,2000);
%  x2=path1(index,1);
% y2=path1(index,2);
% z2=zeros(length(y2),1);
% goal=[100,0];
% X = [x2,y2,z2];
% [L,R2] = curvature(X);
% k=1./R2; 
% 
% % s      =   (hypot(diff(xz(index1,1)),diff(yz(index1,1))));
% % 
% %  select = ~isnan( s );      % Vector of logicals, true at location corresponding
% %                           %   to non-NaN elements of A.
%  s = L ;
%  sf=max(L);                   %total Length
%  vmax=1;                      %maximum reverse velocity
%  amax=1;                      %maximum longitudinal Acceleration
%  dmax=-1;                     %maximum longitudinal deceleration
%  vf=0;                        %final velocity 
%  vi=V_in;                     %Initial Velocity
%  sa=((vmax)^2-(vi)^2)/(2*amax);
%  sb=sf-(((((vf)^2-(vmax)^2)/(2*dmax))));
%  s1=0;
%  
%  V=nan(2000,1);
%  for i=1:length(s)
%    
%     % i=i+1
%     % Vk=sqrt(0.6/abs(k(i)))
%      if k(i)<=max(k)
%           Vk=sqrt(0.6/abs(max(k))); %velocity based on curvature
%       else
%           Vk=vmax;
%       end
%      if (s(i)+(s1))<=sa
%          v=sqrt((2*amax*s(i)+s1)+(vi)^2); %velocity in first phase
% %          if i==1
% %              v=0;
% %             
% %          end
%      elseif (s(i)+(s1))>=sa && (s(i)+(s1))<=sb
%          
%          v=vmax;                           %velocity in 2nd phase
%      else (s(i)+(s1))>=sb && (s(i)+(s1))<=sf;
%          
%          v=sqrt((2*(dmax)*((s(i)+s1)-sb))+(vmax)^2); %velocity in third phase
%      end
%     % s1=s(i)+s1
%      %V4=min(v,2);
%      V(i,1)=-min(Vk,v);
% %     V=[V;V3];
% %      S=[S;s1];
%   
%  end
%  
%  %plot(L,-V*3.6)
% % hold on
% %V=smooth(V,5);
% %path= interparc(0:0.01:1,xz(index1,1),yz(index1,1),V,L,'linear');
% else
    %% Velocity profile for forward path
   dir=1;
 index=find((path1(:,4)==1));
  index2=length(index);
 path=nan(index2*5,3);
 path_tf=nan(1,2000);
 path_input=nan(2000,3);
  Length=nan(1,2000);
 velocity=nan(1,2000);
 x2=path1(index,1);
y2=path1(index,2);
z2=zeros(length(y2),1);
goal=[x2(end,1),y2(end,1)];
%y2 = cos(linspace(0,3*pi));
X = [x2,y2,z2];
[L,R2] = curvature(X);
k=1./R2;
%  %%
% s      =   (hypot(diff(xz(index1,1)),diff(yz(index1,1))));
% 
%  select = ~isnan( s );      % Vector of logicals, true at location corresponding
%                           %   to non-NaN elements of A.
 s = L ;
 sf=max(L);                   %total Length
 vmax=10;                   %maximum forward velocity
 amax=2;                      %maximum longitudinal Acceleration
 dmax=-2;                     %maximum longitudinal deceleration
 vf=0;                        %final velocity 
 vi=V_in;                     %Initial Velocity
 sa=((vmax)^2-(vi)^2)/(2*amax);
  sb=sf-(((((vf)^2-(vmax)^2)/(2*dmax))));

  s1=0;
 

 
 V=nan(2000,1);
 for i=1:length(s)
   
    % i=i+1
    % Vk=sqrt(0.6/abs(k(i)))
     if k(i)<=max(k)
          Vk=sqrt(2/abs(max(k))); %velocity based on curvature
      else
          Vk=vmax;
      end
     if (s(i)+(s1))<=sa
         v=sqrt((2*amax*s(i)+s1)+(vi)^2); %velocity in first phase
%          if i==1
%              v=0;
%             
%          end
     elseif (s(i)+(s1))>=sa && (s(i)+(s1))<=sb
         
         v=vmax;                            %velocity in second phase
     else (s(i)+(s1))>=sb && (s(i)+(s1))<=sf;
         
         v=sqrt((2*(dmax)*((s(i)+s1)-sb))+(vmax)^2); %velocity in third phase
     end
    % s1=s(i)+s1
     V4=min(v,2);
     V(i,1)=min(Vk,v);          %final velocity at each waypoint
%     V=[V;V3];
%      S=[S;s1];
  
 end
%end
select=~isnan(V);
V2=V(select);
%% Intrapolation of the path
k=length(x2)*5;
path(:,1)=pchip(linspace(1,length(x2),length(x2)),x2,linspace(1,length(x2),length(x2)*5));
path(:,2)=pchip(linspace(1,length(y2),length(y2)),y2,linspace(1,length(y2),length(y2)*5));
velocity(1,(1:k))=pchip(linspace(1,length(x2),length(x2)),V2,linspace(1,length(x2),length(x2)*5));
path(:,3)=pchip(linspace(1,length(x2),length(x2)),L,linspace(1,length(x2),length(x2)*5)); 
vel1(1,1:length(V2))=V2;   
path_tf(1,(1:k))=path(:,3);
        j=10;
        d_tot=0; 
        
%% Extrapolation of paths
         while(d_tot<0.8)
            j=j+1;
            extx=interp1(linspace(1,length(path(:,1)),length(path(:,1))),path(:,1),linspace(1,length(path(:,1))+(j),length(path(:,1))+(j)),'linear','extrap');
            exty=interp1(linspace(1,length(path(:,2)),length(path(:,2))),path(:,2),linspace(1,length(path(:,2))+(j),length(path(:,2))+(j)),'linear','extrap');
               
           % extx=extx';
            %exty=exty';
            
            d       =   hypot(diff(extx(length(path(:,1)):length(extx))),diff(exty(length(path(:,2)):length(exty))));
            d_tot   =   sum (d);        % total distance coverd by motion primitives
         end
          j1=length((~isnan(extx)));
         velocity(1,(k-5:j1))=pchip(linspace(1,6,6),velocity(1,(k-5:k)),linspace(1,6,j1-k+6));
  path_tf(1,(k-5:j1))=pchip(linspace(1,6,6),path_tf(1,(k-5:k)),linspace(1,6,j1-k+6));
  path_input((1:j1),1)= extx(1,(1:j1));
  path_input((1:j1),2) = exty(1,(1:j1));% When directon changes simulate 
         path_input(:,3) = zeros(1,length(path_input(:,1)));
         Length(1,(1:k))=path(:,3);
         %path_tf(1,:)=path(:,3)';
end

== matlab function Motion_planner_Street_Drone/Dynamic_Obstacle_avoidance/MATLAB Function2 ==
  data: path input; velocity1 input; new output; dynobst_x output; dynobst_y output; thetad output; Vel_Dyn output; dyn_switch output; x_stop output; y_stop output; id1 output; xa input; ya input; ta input; mode input; id input; id1 input
function [new,dynobst_x,dynobst_y,thetad,Vel_Dyn,dyn_switch,x_stop,y_stop,id1]  = fcn( path,velocity1,xa,ya,ta, mode,id,id1)
coder.extrinsic('InPolygon')
%this function developed for dynamic obstacle detection

%prdefined the variable
Vel_Dyn=nan(1000,2);
dyn_switch=0;
v2=1;
y1=mode;
new=0;
cur =   struct('xa',0,'ya',0);
x_i=xa;
y_i=ya;
t_i=ta;
%vel_in=Vin;

%%slect the nan free Path
select = ~isnan(path(:,1));
path1=path(select,(1:4));
path_inputx=path1(:,1);
path_inputy=path1(:,2);
path_inputtf=path1(:,3);
velocity=velocity1(1,select)';

%% check the dynamic obstacle inside the detection zone
obst_check=0;
% Dynamic obstacle Pose 
 x_dobst=60;
 y_dobst=9;    %0
 t_dobst=270;  %0
thetad=deg2rad(t_dobst);
  cur.xa=xa;
  cur.ya=ya;
  cur.t=ta;
dynobst_x=inf;
dynobst_y=inf;
x_stop=nan(1);
y_stop=nan(1);
dyn_obs_inside_window = check_for_dyn_obs(cur,x_dobst,y_dobst,1);

%% check the collison time
if dyn_obs_inside_window==true && id1~=id
        %disp('obstacle')
       id1=id;
       dyn_switch=0;
       xz=path_inputx;
       yz=path_inputy;
       thetaz=path_inputtf;
       cur.xa=0;
       cur.ya=0;
       
 dist=nan(length(xz)-1,1);
 dist=hypot(diff(xz),diff(yz));
distance=nan(length(xz),1);
distance1=nan(length(xz),1);
 distance=[0;dist];
 for i=1:1:length(distance)
     if i==1
       distance1(i,:)=0;
     else
        distance1(i,:)=distance(i)+distance1(i-1);
     end
 end
 dist1=hypot(path(1,1)-xa,path(1,2)-ya);
 [min_dist,idx11]=min(abs(distance1-dist1)); %find the nearest index in the reference path
 time=nan(length(distance),1);
 Time=nan(length(distance),1);
  for i=idx11:1:length(distance)
      time(i,:)=distance(i,1)/velocity(i,1);
  end
  
% Calculate the time to travel
% time=distance(:,1)/velocity(:,1);
time(isinf(time)) = 0.2;
time(isnan(time)) = 0;
  for i=1:1:length(time)
     if i==1
       Time(i,:)=0;
     else
        Time(i,:)=time(i)+Time(i-1);
     end
  end
 
  dobst_dist=Time*0.5;
  dobsx=x_dobst+(dobst_dist*(cosd(t_dobst)));
  dobsy=y_dobst+(dobst_dist*(sind(t_dobst)));
%   dobsyz=ones(length(Time),1)*dobsy;
%   dobsxz=dobsx+dobst;
 path_input=[xz,yz,thetaz,Time];
 obs_path=[dobsx,dobsy,Time];
% plot(dobsx,dobsy)
 [x1,y1,coll_time,idx]=dynamic_collison(path_input,obs_path,thetad);
collison_time=coll_time
%% 1st approach (stop and go)
if collison_time~=inf
stop_time=path_input(idx,4);
time_to_stop=4;
new_path=nan(length(path_input(:,1))+40,5);
idx1=find((path_input(:,4)<=stop_time));
idx2=find((path_input(:,4)>stop_time));
time_stop=[0.1:0.1:4]';
   x_stop=path_input(idx,1)
  y_stop=path_input(idx,2)
new_path(:,1)=[path_input(idx1,1);ones(length(time_stop),1)*(path_input(idx,1));path_input(idx2,1)];
new_path(:,2)=[path_input(idx1,2);ones(length(time_stop),1)*(path_input(idx,2));path_input(idx2,2)];
new_path(:,3)=[path_input(idx1,3);ones(length(time_stop),1)*(path_input(idx,3));path_input(idx2,3)];
new_path(:,4)=[path_input(idx1,4);ones(length(time_stop),1)*(path_input(idx,4))+time_stop;path_input(idx2,4)+4];

%%
idx1=find((new_path(:,4)<=stop_time));
idx2=find((new_path(:,4)>stop_time));
xz1=new_path(idx1,1);
yz1=new_path(idx1,2);
zdir1=ones(length(xz1),1);

 V1=Velocity_profiler(xz1,yz1,zdir1);

xz2=new_path(idx2,1);
yz2=new_path(idx2,2);
zdir2=ones(length(xz2),1);
 V2=Velocity_profiler(xz2,yz2,zdir2);
 
 %updated velocity profile
 V=[V1;V2];
%  
  dist=nan(length(new_path(:,1))-1,1);
  distance=nan(length(new_path(:,1)),1);
% 
  dist=hypot(diff(new_path(:,1)),diff(new_path(:,2)));
    distance=[0;dist];
%    
     time1=nan(length(distance),1);
  Time1=nan(length(distance),1);
 for i=1:1:length(distance)
      time1(i,:)=distance(i,1)/V(i,1);
 end
  time1(isinf(time1)) = 0.2;
 time1(isnan(time1)) = 0.2;
  for i=1:1:length(time1)
%    
     if i==1
     Time1(i,:)=0;
      else
         Time1(i,:)=time1(i)+Time1(i-1);
      end
  end

Time=new_path(:,4);
path_input=[new_path(:,1),new_path(:,2),new_path(:,3),Time];
  dobst_dist=Time*0.5;
  dobsx=x_dobst+(dobst_dist*(cosd(t_dobst)));
  dobsy=y_dobst+(dobst_dist*(sind(t_dobst)));
 obs_path=[dobsx,dobsy,Time];
 [x1,y1,coll_time,idx3]=dynamic_collison(path_input,obs_path,thetad);
coll_time1=coll_time

if coll_time1==inf
    new=0;
    dyn_switch=-1;
else
    %2nd apprach (replanning)
    new=1;
   dynobst_x=obs_path(idx3,1);
  dynobst_y=obs_path(idx3,2);
  
end

  j=length(V);

Vel_Dyn(1:j,1)=Time1(:,1);
Vel_Dyn(1:j,2)=V(:,1);
end

   

   return

 end    
thetad=t_dobst;

  end

== matlab function Motion_planner_Street_Drone/Trajectory Tracker/ Lateral Controller/Fwd_Controller/MATLAB Function1 ==
  data: data input; u input; y output
function y = fcn(data, u)
if u==-1
    y=data(1);
else
y = data(u);


end
